simulink model "fullSystemModel"  (R2018a)
settings: Solver=ode3  StartTime=0.0  StopTime=1000  FixedStep=1  MinStep=1e-8  RelTol=1e-8
undefined symbols (not defined in the file or in its folder): DiscIntNeverNeededParam
libraries: BupSimulinkLibraries x32, simulink_extras x22, simulink x2, SignalEditorBlockLib x2
(part 1 of 3)
settings Model: PauseTimes=500  PacingRate=5  Creator=Юзер33  LastModifiedBy=User33
settings DataIOCC: SaveFormat=Array  OutputSaveName=P_lon
settings OptimizationCC: DefaultParameterBehavior=Inlined  UseDivisionForNetSlopeComputation=on  UseFloatMulNetSlope=on  InlineInvariantSignals=on  PassReuseOutputArgsAs=Individual arguments  ZeroExternalMemoryAtStartup=off  ZeroInternalMemoryAtStartup=off  NoFixptDivByZeroProtection=on  EfficientFloat2IntCast=on  LifeSpan=1  OptimizationLevel=level1  OptimizationCustomize=off
settings DebuggingCC: ParameterTunabilityLossMsg=error
settings HardwareCC: ProdBitPerPointer=32  ProdBitPerSizeT=32  ProdBitPerPtrDiffT=32  ProdLargestAtomicInteger=Long  ProdLargestAtomicFloat=Double  ProdWordSize=32  ProdHWDeviceType=ARM Compatible->ARM Cortex
settings SFSimCC: MATLABDynamicMemAlloc=off
settings RTWCC: SystemTargetFile=ert.tlc  GenCodeOnly=on  PackageGeneratedCodeAndArtifacts=on  PackageName=BupModel  TemplateMakefile=ert_default_tmf  GenerateReport=on  RTWVerbose=off  RTWUseSimCustomCode=on  BuildConfiguration=Faster Runs  IncludeHyperlinkInReport=on  LaunchReport=on  GenerateTraceInfo=on  GenerateTraceReport=on  GenerateTraceReportSl=on  GenerateTraceReportSf=on  GenerateTraceReportEml=on  GenerateWebview=on  GenerateCodeMetricsReport=on  GenerateCodeReplacementReport=on
settings CodeAppCC: ForceParamTrailComments=on  IgnoreCustomStorageClasses=off  OperatorAnnotations=on  SimulinkDataObjDesc=on  SFDataObjDesc=on  MATLABFcnDesc=on  CustomSymbolStrGlobalVar=rt$N$M  CustomSymbolStrType=$N$M  CustomSymbolStrFcn=$N$M$F  CustomSymbolStrMacro=$N$M  InsertBlockDesc=on  StateflowObjectComments=on  MATLABSourceComments=on  ReqsInCode=on  UseSimReservedNames=on
settings ERTTargetCC: TargetLangStandard=C99 (ISO)  GenerateSampleERTMain=on  IncludeMdlTerminateFcn=off  CombineSignalStateStructs=on  SupportComplex=off  SupportNonInlinedSFcns=on  RemoveResetFunc=off  InlinedParameterPlacement=NonHierarchical  RootIOFormat=Structure reference  ERTCustomFileTemplate=example_file_process.tlc  ERTFilePackagingFormat=CompactWithDataFile  IndentStyle=Allman

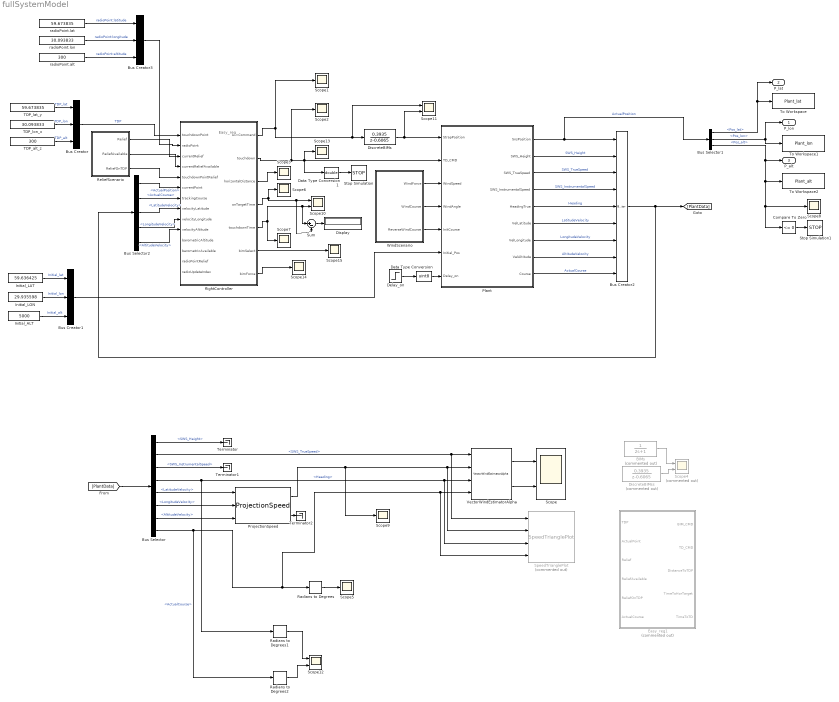
== system fullSystemModel ==
  note: Easy_reg_
  BIMs : TransferFcn  Commented=on  Denominator=[2 1]
  Bus Creator : BusCreator  Inputs=3
  Bus Creator1 : BusCreator  Inputs=3
  Bus Creator2 : BusCreator  Inputs=9
  Bus Creator3 : BusCreator  Inputs=3
  Bus Selector : BusSelector  OutputSignals=SWS_Height,SWS_TrueSpeed,SWS_InstrumentalSpeed,Heading,LatitudeVelocity,LongitudeVelocity,AltitudeVelocity,ActualCourse
  Bus Selector1 : BusSelector  OutputSignals=Pos_lat,Pos_lon,Pos_alt
  Bus Selector2 : BusSelector  OutputSignals=ActualPosition,ActualCourse,LatitudeVelocity,LongitudeVelocity,AltitudeVelocity
  Compare To Zero : simulink/Logic and Bit Operations/Compare To Zero  relop=<=  OutDataTypeStr=boolean
  Data Type Conversion : DataTypeConversion  OutDataTypeStr=uint8
  Data Type Conversion1 : DataTypeConversion  OutDataTypeStr=double
  Delay_on : Step  Time=20  Before=1  SampleTime=0
  DiscreteBIMs : DiscreteTransferFcn  Numerator=[0.3935]  Denominator=[1 -0.6065]
  DiscreteBIMss : DiscreteTransferFcn  Commented=on  Numerator=[0.3935]  Denominator=[1 -0.6065]
  Display : Display
  Easy_reg1 : Subsystem  Commented=on  TreatAsAtomicUnit=on  SystemSampleTime=1
  Initial_ALT : Constant  Value=5000
  Initial_LAT : Constant  Value=59.636425
  Initial_LON : Constant  Value=29.935598
  Plant : Subsystem  TreatAsAtomicUnit=on
  ProjectionSpeed : BupSimulinkLibraries/ProjectionSpeed
  Radians to Degrees : simulink_extras/Transformations/Radians to Degrees
  Radians to Degrees1 : simulink_extras/Transformations/Radians to Degrees
  Radians to Degrees2 : simulink_extras/Transformations/Radians to Degrees
  ReliefScenario : Subsystem  SystemSampleTime=1
  Scope{,10..12} (4 alike) : Scope  NumInputPorts=2
  Scope{1..3,5..9,13..15} (11 alike) : Scope
  Scope4 : Scope  Commented=on  NumInputPorts=2
  SpeedTrianglePlot : BupSimulinkLibraries/SpeedTrianglePlot  Commented=on
  Stop Simulation : Stop
  Stop Simulation1 : Stop
  Sum : Sum  Inputs=|+-
  TDP_alt_z : Constant  Value=300
  TDP_lat_y : Constant  Value=59.673835
  TDP_lon_x : Constant  Value=30.093833
  Terminator : Terminator
  Terminator1 : Terminator
  Terminator2 : Terminator
  To Workspace : ToWorkspace  VariableName=Plant_lat  SaveFormat=Timeseries  SampleTime=-1
  To Workspace1 : ToWorkspace  VariableName=Plant_lon  SaveFormat=Timeseries  SampleTime=-1
  To Workspace2 : ToWorkspace  VariableName=Plant_alt  SaveFormat=Timeseries  SampleTime=-1
  VectorWindEstimatorAlpha : BupSimulinkLibraries/VectorWindEstimatorAlpha  SystemSampleTime=-1
  WindScenario : Subsystem  SystemSampleTime=1
  flightController : Subsystem  TreatAsAtomicUnit=on  SystemSampleTime=1
  radioPoint.alt : Constant  Value=300
  radioPoint.lat : Constant  Value=59.673835
  radioPoint.lon : Constant  Value=30.093833
  P_lon : Outport
  P_lat : Outport  Port=2
  P_alt : Outport  Port=3
  wires:
  TDP_alt_z/1 -> Bus Creator/3  "TDP_alt"
  TDP_lon_x/1 -> Bus Creator/2  "TDP_lon"
  TDP_lat_y/1 -> Bus Creator/1  "TDP_lat"
  Bus Creator/1 -> flightController/1(touchdownPoint)  "TDP"
  Plant/1(SnsPosition) -> Bus Creator2/1, Bus Selector1/1  "ActualPosition"
  Initial_LAT/1 -> Bus Creator1/1  "Initial_lat"
  Initial_LON/1 -> Bus Creator1/2  "Initial_lon"
  Initial_ALT/1 -> Bus Creator1/3  "Initial_alt"
  BIMs/1 -> Scope4/1
  DiscreteBIMss/1 -> Scope4/2
  Bus Selector1/1 -> To Workspace/1, P_lat/1  "<Pos_lat>"
  Delay_on/1 -> Data Type Conversion/1
  DiscreteBIMs/1 -> Plant/1(StrapPosition), Scope11/2
  flightController/1(bimCommand) -> Scope1/1, Scope11/1, DiscreteBIMs/1
  flightController/2(touchdown) -> Scope2/1, Scope13/1, Data Type Conversion1/1, Plant/2(TD_CMD)
  Data Type Conversion/1 -> Plant/7(Delay_on)
  Bus Selector1/2 -> P_lon/1, To Workspace1/1  "<Pos_lon>"
  Bus Selector1/3 -> Scope8/1, Compare To Zero/1, To Workspace2/1, P_alt/1  "<Pos_alt>"
  Plant/7(VelLongitude) -> Bus Creator2/7  "LongitudeVelocity"
  Plant/8(VelAltitude) -> Bus Creator2/8  "AltitudeVelocity"
  Plant/6(VelLatitude) -> Bus Creator2/6  "LatitudeVelocity"
  Plant/2(SWS_Height) -> Bus Creator2/2  "SWS_Height"
  Plant/5(HeadingTrue) -> Bus Creator2/5  "Heading"
  Plant/4(SWS_InstrumentalSpeed) -> Bus Creator2/4  "SWS_InstrumentalSpeed"
  Plant/9(Course) -> Bus Creator2/9  "ActualCourse"
  Plant/3(SWS_TrueSpeed) -> Bus Creator2/3  "SWS_TrueSpeed"
  WindScenario/2(WindCourse) -> Plant/4(WindAngle)
  WindScenario/1(WindForce) -> Plant/3(WindSpeed)
  WindScenario/3(ReverseWindCourse) -> Plant/5(InitCourse)
  [PlantData] -> Bus Selector/1
  Bus Selector/6 -> ProjectionSpeed/2  "<LongitudeVelocity>"
  Bus Selector/2 -> SpeedTrianglePlot/1, VectorWindEstimatorAlpha/1  "<SWS_TrueSpeed>"
  Radians to Degrees/1 -> Scope5/1
  Bus Selector/8 -> Radians to Degrees2/1, SpeedTrianglePlot/4, VectorWindEstimatorAlpha/4, Radians to Degrees/1  "<ActualCourse>"
  Bus Selector/4 -> Radians to Degrees1/1, SpeedTrianglePlot/3, VectorWindEstimatorAlpha/3  "<Heading>"
  VectorWindEstimatorAlpha/1 -> Scope/1
  VectorWindEstimatorAlpha/2 -> Scope/2
  ProjectionSpeed/1 -> Scope9/1, SpeedTrianglePlot/2, VectorWindEstimatorAlpha/2
  Bus Selector/5 -> ProjectionSpeed/1  "<LatitudeVelocity>"
  Bus Selector/7 -> ProjectionSpeed/3  "<AltitudeVelocity>"
  Data Type Conversion1/1 -> Stop Simulation/1
  flightController/3(horizontalDistance) -> Scope3/1
  Compare To Zero/1 -> Stop Simulation1/1
  ReliefScenario/1(Relief) -> flightController/3(currentRelief)
  ReliefScenario/2(ReliefAvailable) -> flightController/4(currentReliefAvailable)
  ReliefScenario/3(ReliefOnTDP) -> flightController/5(touchdownPointRelief)
  Bus Creator2/1 -> Bus Selector2/1, [PlantData]
  Bus Selector2/1 -> flightController/6(currentPoint)  "<ActualPosition>"
  Bus Selector2/2 -> flightController/7(trackingCourse)  "<ActualCourse>"
  Bus Selector2/3 -> flightController/8(velocityLatitude)  "<LatitudeVelocity>"
  Bus Selector2/4 -> flightController/9(velocityLongitude)  "<LongitudeVelocity>"
  Bus Selector2/5 -> flightController/10(velocityAltitude)  "<AltitudeVelocity>"
  Bus Creator1/1 -> Plant/6(Initial_Pos)
  flightController/5(touchdownTime) -> Sum/1, Scope10/2, Scope7/1
  flightController/4(onTargetTime) -> Scope6/1, Sum/2, Scope10/1
  Bus Selector/1 -> Terminator/1  "<SWS_Height>"
  Bus Selector/3 -> Terminator1/1  "<SWS_InstrumentalSpeed>"
  ProjectionSpeed/2 -> Terminator2/1
  Sum/1 -> Display/1
  Radians to Degrees1/1 -> Scope12/1
  Radians to Degrees2/1 -> Scope12/2
  flightController/7(bimForce) -> Scope14/1
  flightController/6(bimSelect) -> Scope15/1
  radioPoint.lon/1 -> Bus Creator3/2  "radioPoint:longitude"
  radioPoint.alt/1 -> Bus Creator3/3  "radioPoint:altitude"
  radioPoint.lat/1 -> Bus Creator3/1  "radioPoint:latitude"
  Bus Creator3/1 -> flightController/2(radioPoint)

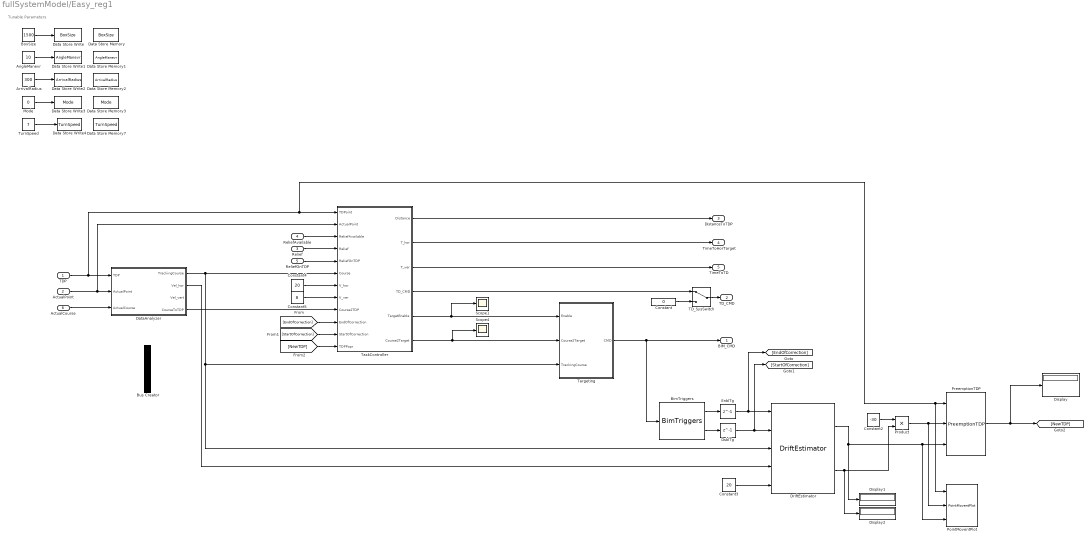
== system fullSystemModel/Easy_reg1 ==
  note: Tunable Parameters
  TDP : Inport
  ActualPoint : Inport  Port=2
  Relief : Inport  Port=3
  ReliefAvailable : Inport  Port=4
  ReliefOnTDP : Inport  Port=5
  ActualCourse : Inport  Port=6
  AngleManevr : Constant  Value=10
  ArrivalRadius : Constant  Value=300
  BimTriggers : BupSimulinkLibraries/BimTriggers
  BoxSize : Constant  Value=1500
  Bus Creator : BusCreator  Inputs=6
  Constant : Constant  Value=0
  Constant2 : Constant  Value=-30
  Constant3 : Constant  Value=20
  Constant4 : Constant  Value=20
  Constant5 : Constant  Value=8
  Data Store Memory : DataStoreMemory  DataStoreName=BoxSize  ReadBeforeWriteMsg=warning  WriteAfterWriteMsg=warning  WriteAfterReadMsg=warning  ShowAdditionalParam=off  OutDataTypeStr=double  Dimensions=1
  Data Store Memory1 : DataStoreMemory  DataStoreName=AngleManevr  ReadBeforeWriteMsg=warning  WriteAfterWriteMsg=warning  WriteAfterReadMsg=warning  ShowAdditionalParam=off  OutDataTypeStr=double  Dimensions=1
  Data Store Memory2 : DataStoreMemory  DataStoreName=ArrivalRadius  ReadBeforeWriteMsg=warning  WriteAfterWriteMsg=warning  WriteAfterReadMsg=warning  ShowAdditionalParam=off  OutDataTypeStr=double  Dimensions=1
  Data Store Memory3 : DataStoreMemory  DataStoreName=Mode  ReadBeforeWriteMsg=warning  WriteAfterWriteMsg=warning  WriteAfterReadMsg=warning  ShowAdditionalParam=off  OutDataTypeStr=uint8  Dimensions=1
  Data Store Memory7 : DataStoreMemory  DataStoreName=TurnSpeed  ReadBeforeWriteMsg=warning  WriteAfterWriteMsg=warning  WriteAfterReadMsg=warning  ShowAdditionalParam=off  OutDataTypeStr=double  Dimensions=1
  Data Store Write : DataStoreWrite  DataStoreName=BoxSize
  Data Store Write1 : DataStoreWrite  DataStoreName=AngleManevr
  Data Store Write2 : DataStoreWrite  DataStoreName=ArrivalRadius
  Data Store Write3 : DataStoreWrite  DataStoreName=Mode
  Data Store Write4 : DataStoreWrite  DataStoreName=TurnSpeed
  DataAnalyzer : Subsystem
  Display : Display
  Display1 : Display
  Display2 : Display
  DriftEstimator : BupSimulinkLibraries/DriftEstimator
  DsblTg : Delay  DelayLength=1  InitialCondition=0
  EnblTg : Delay  DelayLength=1  InitialCondition=0
  Mode : Constant  Value=0  OutDataTypeStr=uint8
  PointMoventPlot : BupSimulinkLibraries/PointMoventPlot
  PreemptionTDP : BupSimulinkLibraries/PreemptionTDP
  Product : Product
  Scope1 : Scope
  Scope4 : Scope
  TD_SysSwitch : ManualSwitch
  Targeting : Subsystem
  TaskController : Stateflow chart  TreatAsAtomicUnit=on  SystemSampleTime=1
  TurnSpeed : Constant  Value=7  OutDataTypeStr=double
  BIM_CMD : Outport
  TD_CMD : Outport  Port=2  OutDataTypeStr=uint8
  DistanceToTDP : Outport  Port=3
  TimeToHorTarget : Outport  Port=4
  TimeToTD : Outport  Port=5
  wires:
  TaskController/4(TD_CMD) -> TD_SysSwitch/1
  BoxSize/1 -> Data Store Write/1
  AngleManevr/1 -> Data Store Write1/1
  ArrivalRadius/1 -> Data Store Write2/1
  TD_SysSwitch/1 -> TD_CMD/1
  Constant/1 -> TD_SysSwitch/2
  Mode/1 -> Data Store Write3/1
  TurnSpeed/1 -> Data Store Write4/1
  TaskController/5(TargetEnable) -> Scope1/1, Targeting/1(Enable)
  DataAnalyzer/2(Vel_hor) -> DriftEstimator/4
  ActualCourse/1 -> DataAnalyzer/3(ActualCourse)
  ReliefAvailable/1 -> TaskController/3(ReliefAvailable)
  Relief/1 -> TaskController/4(Relief)
  ReliefOnTDP/1 -> TaskController/5(ReliefOnTDP)
  TaskController/1(Distance) -> DistanceToTDP/1
  TaskController/2(T_hor) -> TimeToHorTarget/1
  TaskController/3(T_ver) -> TimeToTD/1
  ActualPoint/1 -> DataAnalyzer/2(ActualPoint), TaskController/2(ActualPoint)
  TaskController/6(Course2Target) -> Targeting/2(Course2Target), Scope4/1
  Targeting/1(CMD) -> BimTriggers/1, BIM_CMD/1
  BimTriggers/2 -> DsblTg/1
  DataAnalyzer/1(TrackingCourse) -> DriftEstimator/3, Targeting/3(TrackingCourse), TaskController/6(Course)
  DataAnalyzer/4(CourseToTDP) -> TaskController/9(Course2TDP)
  BimTriggers/1 -> EnblTg/1
  Constant2/1 -> Product/1
  TDP/1 -> PointMoventPlot/1, PreemptionTDP/1, TaskController/1(TDPoint), DataAnalyzer/1(TDP)
  Product/1 -> PointMoventPlot/2, PreemptionTDP/2
  DriftEstimator/2 -> Display2/1, Product/2
  DriftEstimator/1 -> Display1/1, PointMoventPlot/3, PreemptionTDP/3
  EnblTg/1 -> [EndOfCorrection], DriftEstimator/1
  DsblTg/1 -> [StartOfCorrection], DriftEstimator/2
  Constant3/1 -> DriftEstimator/5
  Constant5/1 -> TaskController/8(V_ver)
  Constant4/1 -> TaskController/7(V_hor)
  PreemptionTDP/1 -> [NewTDP], Display/1
  [EndOfCorrection] -> TaskController/10(EndOfCorrection)
  [NewTDP] -> TaskController/12(TDPPopr)
  [StartOfCorrection] -> TaskController/11(StartOfCorrection)

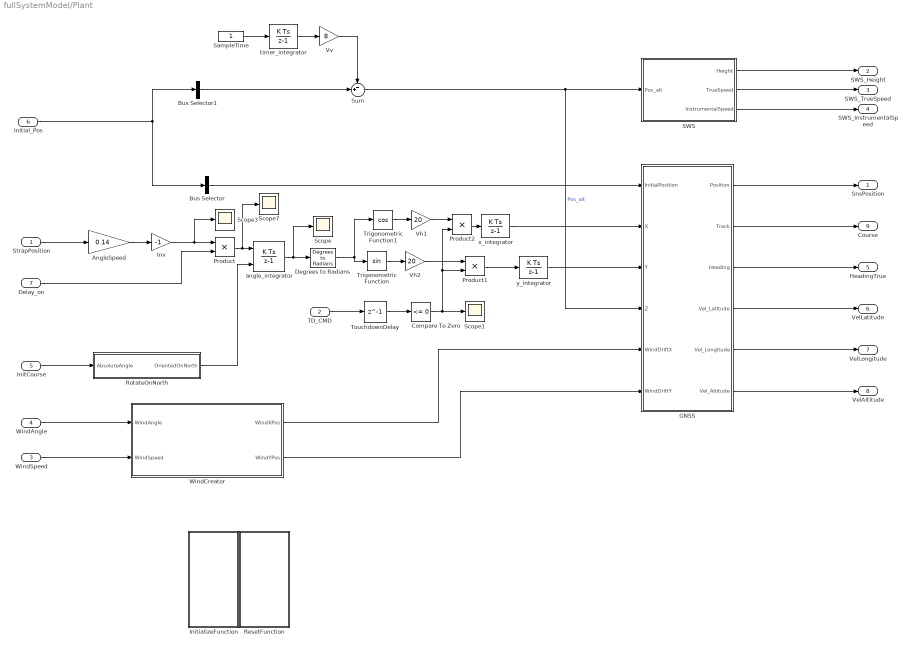
== system fullSystemModel/Plant ==
  StrapPosition : Inport  OutDataTypeStr=double  PortDimensions=1
  TD_CMD : Inport  Port=2  OutDataTypeStr=uint8  PortDimensions=1
  WindSpeed : Inport  Port=3
  WindAngle : Inport  Port=4
  InitCourse : Inport  Port=5
  Initial_Pos : Inport  Port=6
  Delay_on : Inport  Port=7
  AngleSpeed : Gain  Gain=0.14
  Bus Selector : BusSelector  OutputSignals=Initial_lat,Initial_lon  OutputAsBus=on
  Bus Selector1 : BusSelector  OutputSignals=Initial_alt  OutputAsBus=on
  Compare To Zero : simulink/Logic and Bit Operations/Compare To Zero  relop=<=  OutDataTypeStr=boolean
  Degrees to Radians : simulink_extras/Transformations/Degrees to Radians
  GNSS : Subsystem
  InitializeFunction : Subsystem  TreatAsAtomicUnit=on
  Inv : Gain  Gain=-1
  Product : Product
  Product1 : Product
  Product2 : Product
  ResetFunction : Subsystem  TreatAsAtomicUnit=on
  RotateOnNorth : Subsystem
  SWS : Subsystem
  SampleTime : Constant
  Scope{,1,3,7} (4 alike) : Scope
  Sum : Sum  Inputs=-+|
  TouchdownDelay : Delay  DelayLength=1  InitialCondition=0
  Trigonometric Function : Trigonometry
  Trigonometric Function1 : Trigonometry  Operator=cos
  Vh1 : Gain  Gain=20
  Vh2 : Gain  Gain=20
  Vv : Gain  Gain=8
  WindCreator : Subsystem
  angle_integrator : DiscreteIntegrator  InitialConditionSource=external  InitialCondition=90  SampleTime=-1  ICPrevOutput=DiscIntNeverNeededParam  ICPrevScaledInput=DiscIntNeverNeededParam
  timer_integrator : DiscreteIntegrator  SampleTime=-1  ICPrevOutput=DiscIntNeverNeededParam  ICPrevScaledInput=DiscIntNeverNeededParam
  x_integrator : DiscreteIntegrator  SampleTime=-1  ICPrevOutput=DiscIntNeverNeededParam  ICPrevScaledInput=DiscIntNeverNeededParam
  y_integrator : DiscreteIntegrator  SampleTime=-1  ICPrevOutput=DiscIntNeverNeededParam  ICPrevScaledInput=DiscIntNeverNeededParam
  SnsPosition : Outport
  SWS_Height : Outport  Port=2
  SWS_TrueSpeed : Outport  Port=3
  SWS_InstrumentalSpeed : Outport  Port=4
  HeadingTrue : Outport  Port=5
  VelLatitude : Outport  Port=6
  VelLongitude : Outport  Port=7
  VelAltitude : Outport  Port=8
  Course : Outport  Port=9
  wires:
  Degrees to Radians/1 -> Trigonometric Function1/1, Trigonometric Function/1
  angle_integrator/1 -> Scope/1, Degrees to Radians/1
  Trigonometric Function1/1 -> Vh1/1
  Trigonometric Function/1 -> Vh2/1
  Inv/1 -> Product/1, Scope3/1
  Delay_on/1 -> Product/2
  timer_integrator/1 -> Vv/1
  Vv/1 -> Sum/1
  Sum/1 -> GNSS/4(Z), SWS/1(Pos_alt)  "Pos_alt"
  Initial_Pos/1 -> Bus Selector1/1, Bus Selector/1
  Bus Selector/1 -> GNSS/1(InitialPosition)
  Bus Selector1/1 -> Sum/2
  StrapPosition/1 -> AngleSpeed/1
  Product/1 -> Scope7/1, angle_integrator/1
  AngleSpeed/1 -> Inv/1
  SWS/1(Height) -> SWS_Height/1
  SWS/2(TrueSpeed) -> SWS_TrueSpeed/1
  SWS/3(InstrumentalSpeed) -> SWS_InstrumentalSpeed/1
  SampleTime/1 -> timer_integrator/1
  InitCourse/1 -> RotateOnNorth/1(AbsoluteAngle)
  TD_CMD/1 -> TouchdownDelay/1
  WindAngle/1 -> WindCreator/1(WindAngle)
  WindSpeed/1 -> WindCreator/2(WindSpeed)
  RotateOnNorth/1(OrientedOnNorth) -> angle_integrator/2
  x_integrator/1 -> GNSS/2(X)
  y_integrator/1 -> GNSS/3(Y)
  WindCreator/1(WindXPos) -> GNSS/5(WindDriftX)
  WindCreator/2(WindYPos) -> GNSS/6(WindDriftY)
  GNSS/1(Position) -> SnsPosition/1
  GNSS/3(Heading) -> HeadingTrue/1
  GNSS/2(Track) -> Course/1
  GNSS/4(Vel_Latitude) -> VelLatitude/1
  GNSS/5(Vel_Longitude) -> VelLongitude/1
  GNSS/6(Vel_Altitude) -> VelAltitude/1
  Vh1/1 -> Product2/1
  Vh2/1 -> Product1/1
  TouchdownDelay/1 -> Compare To Zero/1
  Compare To Zero/1 -> Product2/2, Product1/2, Scope1/1
  Product1/1 -> y_integrator/1
  Product2/1 -> x_integrator/1

== system fullSystemModel/ReliefScenario ==
  AutoModeA : ManualSwitch  CurrentSetting=0
  AutoModeR : ManualSwitch  CurrentSetting=0
  ReliefAvailableValue : Constant  OutDataTypeStr=uint8
  ReliefOnTDPValue : Constant  Value=100  OutDataTypeStr=int16
  ReliefValue : Constant  Value=100  OutDataTypeStr=int16
  Scope{,1..3} (4 alike) : Scope
  SignalEditor : SignalEditorBlockLib/Signal Editor  FileName=ReliefScenario.mat  ActiveScenario=Scenario  ActiveSignal=ReliefAvailable  IsBus=off  OutputBusObjectStr=Bus: BusObject  SampleTime=1  Interpolate=off  ZeroCross=off  OutputAfterFinalValue=Setting to zero  Unit=inherit
  Relief : Outport
  ReliefAvailable : Outport  Port=2
  ReliefOnTDP : Outport  Port=3
  wires:
  SignalEditor/2 -> Scope1/1, AutoModeA/1
  SignalEditor/1 -> Scope/1, AutoModeR/1
  ReliefAvailableValue/1 -> AutoModeA/2
  ReliefValue/1 -> AutoModeR/2
  AutoModeR/1 -> Scope2/1, Relief/1
  AutoModeA/1 -> Scope3/1, ReliefAvailable/1
  ReliefOnTDPValue/1 -> ReliefOnTDP/1

== system fullSystemModel/WindScenario ==
  AutoModeA : ManualSwitch
  AutoModeS : ManualSwitch
  Constant : Constant  Value=180
  Constant1 : Constant  Value=0
  Degrees to Radians : simulink_extras/Transformations/Degrees to Radians
  Manual Switch : ManualSwitch  CurrentSetting=0
  Scope1 : Scope
  Scope2 : Scope
  Scope3 : Scope
  SignalEditor : SignalEditorBlockLib/Signal Editor  FileName=WindScenario.mat  ActiveScenario=Scenario  ActiveSignal=WindHeading  IsBus=off  OutputBusObjectStr=Bus: BusObject  SampleTime=1  ZeroCross=off  OutputAfterFinalValue=Setting to zero  Unit=inherit
  Sum : Sum  Inputs=++|
  WindAngle : Constant  Value=0
  WindSpeed : Constant  Value=0
  WindForce : Outport
  WindCourse : Outport  Port=2
  ReverseWindCourse : Outport  Port=3
  wires:
  SignalEditor/1 -> AutoModeS/1, Scope2/1
  WindAngle/1 -> AutoModeA/2
  WindSpeed/1 -> AutoModeS/2
  AutoModeS/1 -> WindForce/1
  AutoModeA/1 -> WindCourse/1, Sum/2
  Sum/1 -> Manual Switch/1
  Constant/1 -> Sum/1
  Manual Switch/1 -> ReverseWindCourse/1
  Constant1/1 -> Manual Switch/2
  SignalEditor/2 -> AutoModeA/1, Scope3/1, Degrees to Radians/1
  Degrees to Radians/1 -> Scope1/1

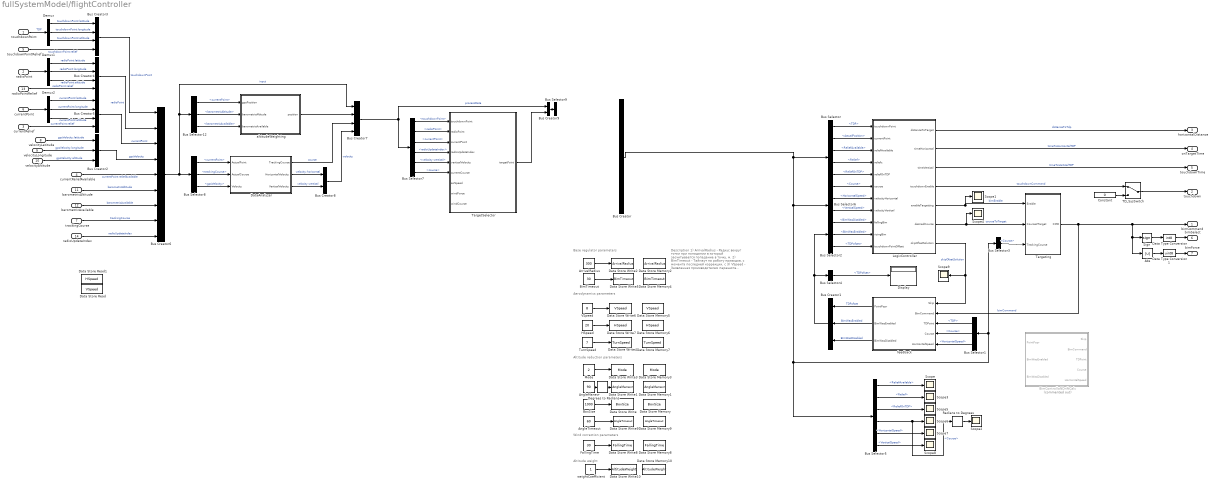
== system fullSystemModel/flightController ==
  note: Altitude weight
  note: Description
      | 1) ArrivalRadius - Радиус вокруг
      | точки при попадании в который
      | засчитывается попадание в
      | точку, м.
      | 2) BimTimeout - Таймаут на работу
      | приводов, с момента последней
      | коррекции, с
      |
      |
      | 3) VSpeed - Заявленная
      | производителем парашюта
      | вертикальная скорость снижения
      | парашюта, м/с.
      | 4) HSpeed - Заявленная
      | производителем парашюта
      | горизонтальная скорость движения
      | парашюта, м/с.
      | 5) TurnSpeed - Заявленная
      | производителем парашюта
      | скорость разворота при 50%
      | затяжке стропы, град/с.
      |
      |
      | 6) Mode - Режим работы
      | регулятора.
      |
      | 7) AngleManevr - Угол отклонения
      | от заданного курса при работе
      | регулятора в
      | режиме углового манёвра, град.
      |
      | 8) BoxSize - Размер коробки в
      | режиме работы 1-Box, м.
      |
      | 9) AngleTimeout - Таймаут между
      | шагами алгоритма потери высоты
      | в режиме работы 3-Angle, сек.
      |
      | 10) FallingTime - Расчетное время
      | между введением посадочной
      | системы в действие и посадкой,
      | сек.
      |
      | 11) Весовой коэффициент
      | для определения высоты (0...1):
      | = 1 Если доверяем только высоте
      | со спутника;
      | = 0 Если доверяем только
      | барометрической высоте;
  note: Altitude reduction parameters
  note: Aerodynamics parameters
  note: Base regulator parameters
  note: Wind correction parameters
  touchdownPoint : Inport
  radioPoint : Inport  Port=2  PortDimensions=3
  currentRelief : Inport  Port=3
  currentReliefAvailable : Inport  Port=4
  touchdownPointRelief : Inport  Port=5
  currentPoint : Inport  Port=6
  trackingCourse : Inport  Port=7
  velocityLatitude : Inport  Port=8
  velocityLongitude : Inport  Port=9
  velocityAltitude : Inport  Port=10
  barometricAltitude : Inport  Port=11
  barometricAvailable : Inport  Port=12
  radioPointRelief : Inport  Port=13
  radioUpdateIndex : Inport  Port=14
  Abs : Abs
  AngleManevr : Constant  Value=90
  AngleTimeout : Constant  Value=60  OutDataTypeStr=uint32
  ArrivalRadius : Constant  Value=300
  BimControllaNDriftCalc : Subsystem  Commented=on
  BimTimeout : Constant  Value=30  OutDataTypeStr=uint32
  BoxSize : Constant  Value=1000
  Bus Creator : BusCreator  Inputs=10
  Bus Creator1 : BusCreator  Inputs=3
  Bus Creator2 : BusCreator  Inputs=3
  Bus Creator{3..5,7} (4 alike) : BusCreator  Inputs=4
  Bus Creator6 : BusCreator  Inputs=9
  Bus Creator8 : BusCreator  Inputs=2
  Bus Creator9 : BusCreator  Inputs=2
  Bus Selector : BusSelector  OutputSignals=TDP,ActualPosition,ReliefAvailable,Relief,ReliefOnTDP,Course
  Bus Selector1 : BusSelector  OutputSignals=TDP,Course,HorizontalSpeed
  Bus Selector12 : BusSelector  OutputSignals=currentPoint,barometricAltitude,barometricAvailable
  Bus Selector2 : BusSelector  OutputSignals=BimWasDisabled,BimWasEnabled,TDPofset
  Bus Selector3 : BusSelector  OutputSignals=Course
  Bus Selector4 : BusSelector  OutputSignals=TDPofset
  Bus Selector5 : BusSelector  OutputSignals=ReliefAvailable,Relief,ReliefOnTDP,Course,HorizontalSpeed,VerticalSpeed
  Bus Selector6 : BusSelector  OutputSignals=HorizontalSpeed,VerticalSpeed
  Bus Selector7 : BusSelector  OutputSignals=input.touchdownPoint,input.radioPoint,currentPoint,input.radioUpdateIndex,velocity.velocity:vertical,course
  Bus Selector8 : BusSelector  OutputSignals=currentPoint,trackingCourse,gpsVelocity
  Bus Selector9 : BusSelector  OutputSignals=processData.currentPoint,targetPoint,processData.course,processData.velocity,processData.input.currentPoint:reliefAvailable  OutputAsBus=on
  Constant : Constant  Value=0
  Data Store Memory : DataStoreMemory  DataStoreName=BoxSize  ReadBeforeWriteMsg=warning  WriteAfterWriteMsg=warning  WriteAfterReadMsg=warning  ShowAdditionalParam=off  OutDataTypeStr=double  Dimensions=1
  Data Store Memory1 : DataStoreMemory  DataStoreName=AngleManevr  ReadBeforeWriteMsg=warning  WriteAfterWriteMsg=warning  WriteAfterReadMsg=warning  ShowAdditionalParam=off  OutDataTypeStr=double  Dimensions=1
  Data Store Memory10 : DataStoreMemory  DataStoreName=AltitudeWeight  ReadBeforeWriteMsg=warning  WriteAfterWriteMsg=warning  WriteAfterReadMsg=warning  ShowAdditionalParam=off  OutDataTypeStr=double  Dimensions=1
  Data Store Memory2 : DataStoreMemory  DataStoreName=ArrivalRadius  ReadBeforeWriteMsg=warning  WriteAfterWriteMsg=warning  WriteAfterReadMsg=warning  ShowAdditionalParam=off  OutDataTypeStr=double  Dimensions=1
  Data Store Memory3 : DataStoreMemory  DataStoreName=Mode  ReadBeforeWriteMsg=warning  WriteAfterWriteMsg=warning  WriteAfterReadMsg=warning  ShowAdditionalParam=off  OutDataTypeStr=uint8  Dimensions=1
  Data Store Memory4 : DataStoreMemory  DataStoreName=BimTimeout  ReadBeforeWriteMsg=warning  WriteAfterWriteMsg=warning  WriteAfterReadMsg=warning  ShowAdditionalParam=off  OutDataTypeStr=uint32  Dimensions=1
  Data Store Memory5 : DataStoreMemory  DataStoreName=VSpeed  ReadBeforeWriteMsg=warning  WriteAfterWriteMsg=warning  WriteAfterReadMsg=warning  ShowAdditionalParam=off  OutDataTypeStr=double  Dimensions=1
  Data Store Memory6 : DataStoreMemory  DataStoreName=HSpeed  ReadBeforeWriteMsg=warning  WriteAfterWriteMsg=warning  WriteAfterReadMsg=warning  ShowAdditionalParam=off  OutDataTypeStr=double  Dimensions=1
  Data Store Memory7 : DataStoreMemory  DataStoreName=TurnSpeed  ReadBeforeWriteMsg=warning  WriteAfterWriteMsg=warning  WriteAfterReadMsg=warning  ShowAdditionalParam=off  OutDataTypeStr=double  Dimensions=1
  Data Store Memory8 : DataStoreMemory  DataStoreName=FallingTime  ReadBeforeWriteMsg=warning  WriteAfterWriteMsg=warning  WriteAfterReadMsg=warning  ShowAdditionalParam=off  OutDataTypeStr=double  Dimensions=1
  Data Store Memory9 : DataStoreMemory  DataStoreName=AngleTimeout  ReadBeforeWriteMsg=warning  WriteAfterWriteMsg=warning  WriteAfterReadMsg=warning  ShowAdditionalParam=off  OutDataTypeStr=uint32  Dimensions=1
  Data Store Read : DataStoreRead  DataStoreName=VSpeed
  Data Store Read1 : DataStoreRead  DataStoreName=HSpeed
  Data Store Write : DataStoreWrite  DataStoreName=BoxSize
  Data Store Write1 : DataStoreWrite  DataStoreName=AngleManevr
  Data Store Write10 : DataStoreWrite  DataStoreName=AltitudeWeight
  Data Store Write2 : DataStoreWrite  DataStoreName=ArrivalRadius
  Data Store Write3 : DataStoreWrite  DataStoreName=Mode
  Data Store Write4 : DataStoreWrite  DataStoreName=TurnSpeed
  Data Store Write5 : DataStoreWrite  DataStoreName=BimTimeout
  Data Store Write6 : DataStoreWrite  DataStoreName=VSpeed
  Data Store Write7 : DataStoreWrite  DataStoreName=HSpeed
  Data Store Write8 : DataStoreWrite  DataStoreName=FallingTime
  Data Store Write9 : DataStoreWrite  DataStoreName=AngleTimeout
  Data Type Conversion : DataTypeConversion  OutDataTypeStr=int8
  Data Type Conversion1 : DataTypeConversion  OutDataTypeStr=uint8
  DataAnalyzer : Subsystem
  Degrees to Radians : simulink_extras/Transformations/Degrees to Radians
  Demux : Demux  Outputs=3
  Demux1 : Demux  Outputs=3
  Demux2 : Demux  Outputs=3
  Display : Display
  FallingTime : Constant  Value=30
  HSpeed : Constant  Value=20
  LogicController : Stateflow chart  TreatAsAtomicUnit=on  SystemSampleTime=1
  Mode : Constant  Value=2  OutDataTypeStr=uint8
  Radians to Degrees : simulink_extras/Transformations/Radians to Degrees
  Scope{,1..9} (10 alike) : Scope
  Sign : Signum
  TD_SysSwitch : ManualSwitch
  TargetSelector : Stateflow chart  TreatAsAtomicUnit=on
  Targeting : Subsystem
  TurnSpeed : Constant  Value=7  OutDataTypeStr=double
  VSpeed : Constant  Value=8
  altitudeWeighting : Subsystem
  feedback : Subsystem
  weightCoefficient : Constant  OutMin=[0]  OutMax=[1]  OutDataTypeStr=double
  bimCommand : Outport
  touchdown : Outport  Port=2  OutDataTypeStr=uint8
  horizontalDistance : Outport  Port=3
  onTargetTime : Outport  Port=4
  touchdownTime : Outport  Port=5
  bimSelect : Outport  Port=6  OutDataTypeStr=int8
  bimForce : Outport  Port=7  OutDataTypeStr=uint8
  wires:
  LogicController/4(touchdownEnable) -> TD_SysSwitch/1  "touchdownCommand"
  BoxSize/1 -> Data Store Write/1
  AngleManevr/1 -> Degrees to Radians/1
  ArrivalRadius/1 -> Data Store Write2/1
  TD_SysSwitch/1 -> touchdown/1
  Constant/1 -> TD_SysSwitch/2
  Mode/1 -> Data Store Write3/1
  TurnSpeed/1 -> Data Store Write4/1
  LogicController/5(enableTargetting) -> Scope1/1, Targeting/1(Enable)  "bimEnable"
  LogicController/1(distanceToTarget) -> horizontalDistance/1  "distanceToTdp"
  LogicController/2(timeHorizontal) -> onTargetTime/1  "timeToHorizontalTDP"
  LogicController/3(timeVertical) -> touchdownTime/1  "timeToVerticalTDP"
  LogicController/6(desiredCourse) -> Scope4/1, Targeting/2(Course2Target)  "courseToTarget"
  Targeting/1(CMD) -> feedback/2(BimCommand), bimCommand/1, Abs/1, Sign/1  "bimCommand"
  Bus Selector/2 -> LogicController/2(currentPoint)  "<ActualPosition>"
  Bus Selector/3 -> LogicController/3(reliefAvailable)  "<ReliefAvailable>"
  Bus Selector/4 -> LogicController/4(reliefc)  "<Relief>"
  Bus Selector/5 -> LogicController/5(reliefOnTDP)  "<ReliefOnTDP>"
  Bus Selector/6 -> LogicController/6(course)  "<Course>"
  Bus Selector1/1 -> feedback/3(TDPoint)  "<TDP>"
  Bus Selector1/2 -> feedback/4(Course)  "<Course>"
  Bus Selector1/3 -> feedback/5(HorizontalSpeed)  "<HorizontalSpeed>"
  feedback/2(BimWasEnabled) -> Bus Creator1/2  "BimWasEnabled"
  feedback/3(BimWasDisabled) -> Bus Creator1/3  "BimWasDisabled"
  Bus Creator1/1 -> Bus Selector2/1, Bus Selector4/1
  Bus Selector2/1 -> LogicController/9(fallingBim)  "<BimWasDisabled>"
  Bus Selector2/2 -> LogicController/10(risingBim)  "<BimWasEnabled>"
  Bus Selector2/3 -> LogicController/11(touchdownPointOffset)  "<TDPofset>"
  Bus Selector3/1 -> Targeting/3(TrackingCourse)  "<Course>"
  feedback/1(PointPopr) -> Bus Creator1/1  "TDPofset"
  Bus Selector/1 -> LogicController/1(touchdownPoint)  "<TDP>"
  BimTimeout/1 -> Data Store Write5/1
  VSpeed/1 -> Data Store Write6/1
  HSpeed/1 -> Data Store Write7/1
  FallingTime/1 -> Data Store Write8/1
  Bus Selector4/1 -> Display/1  "<TDPofset>"
  Bus Creator/1 -> Bus Selector5/1, Bus Selector3/1, Bus Selector1/1, Bus Selector6/1, Bus Selector/1
  Bus Selector5/1 -> Scope/1  "<ReliefAvailable>"
  Bus Selector5/2 -> Scope3/1  "<Relief>"
  Bus Selector5/3 -> Scope5/1  "<ReliefOnTDP>"
  Bus Selector5/4 -> Radians to Degrees/1, Scope6/1  "<Course>"
  Bus Selector5/5 -> Scope7/1  "<HorizontalSpeed>"
  Bus Selector5/6 -> Scope8/1  "<VerticalSpeed>"
  AngleTimeout/1 -> Data Store Write9/1
  Degrees to Radians/1 -> Data Store Write1/1
  LogicController/7(skipOfsetSolution) -> feedback/1(Skip), Scope9/1  "skipOfsetSolution"
  Bus Selector6/1 -> LogicController/7(velocityHorizontal)  "<HorizontalSpeed>"
  Bus Selector6/2 -> LogicController/8(velocityVertical)  "<VerticalSpeed>"
  Sign/1 -> Data Type Conversion/1
  Abs/1 -> Data Type Conversion1/1
  Radians to Degrees/1 -> Scope2/1
  weightCoefficient/1 -> Data Store Write10/1
  Data Type Conversion/1 -> bimSelect/1
  Data Type Conversion1/1 -> bimForce/1
  touchdownPoint/1 -> Demux/1  "TDP"
  Demux/1 -> Bus Creator3/1  "touchdownPoint:latitude"
  Demux/2 -> Bus Creator3/2  "touchdownPoint:longitude"
  Demux/3 -> Bus Creator3/3  "touchdownPoint:atlitude"
  touchdownPointRelief/1 -> Bus Creator3/4  "touchdownPoint:relief"
  radioPoint/1 -> Demux1/1
  radioPointRelief/1 -> Bus Creator4/4  "radioPoint:relief"
  Demux1/3 -> Bus Creator4/3  "radioPoint:altitude"
  Demux1/2 -> Bus Creator4/2  "radioPoint:longitude"
  Demux1/1 -> Bus Creator4/1  "radioPoint:latitude"
  Demux2/3 -> Bus Creator5/3  "currentPoint:altitude"
  currentPoint/1 -> Demux2/1
  currentRelief/1 -> Bus Creator5/4  "currentPoint:relief"
  velocityLatitude/1 -> Bus Creator2/1  "gpsVelocity:latitude"
  velocityLongitude/1 -> Bus Creator2/2  "gpsVelocity:longitude"
  velocityAltitude/1 -> Bus Creator2/3  "gpsVelocity:altitude"
  Bus Creator3/1 -> Bus Creator6/1  "touchdownPoint"
  Bus Creator4/1 -> Bus Creator6/2  "radioPoint"
  Bus Creator5/1 -> Bus Creator6/3  "currentPoint"
  Bus Creator2/1 -> Bus Creator6/4  "gpsVelocity"
  currentReliefAvailable/1 -> Bus Creator6/5  "currentPoint:reliefAvailable"
  trackingCourse/1 -> Bus Creator6/8  "trackingCourse"
  barometricAltitude/1 -> Bus Creator6/6  "barometricAltitude"
  barometricAvailable/1 -> Bus Creator6/7  "barometricAvailable"
  Bus Selector8/1 -> DataAnalyzer/1(ActualPoint)  "<currentPoint>"
  Bus Selector8/2 -> DataAnalyzer/2(ActualCourse)  "<trackingCourse>"
  Bus Creator6/1 -> Bus Creator7/1, Bus Selector12/1, Bus Selector8/1  "input"
  Bus Selector8/3 -> DataAnalyzer/3(Velocity)  "<gpsVelocity>"
  Bus Selector12/1 -> altitudeWeighting/1(gpsPosition)  "<currentPoint>"
  Bus Selector12/2 -> altitudeWeighting/2(barometricAltitude)  "<barometricAltitude>"
  Bus Selector12/3 -> altitudeWeighting/3(barometricAvailable)  "<barometricAvailable>"
  radioUpdateIndex/1 -> Bus Creator6/9  "radioUpdateIndex"
  DataAnalyzer/2(HorizontalVelocity) -> Bus Creator8/1  "velocity:horizontal"
  DataAnalyzer/3(VerticalVelocity) -> Bus Creator8/2  "velocity:vertical"
  Bus Creator8/1 -> Bus Creator7/4  "velocity"
  DataAnalyzer/1(TrackingCourse) -> Bus Creator7/3  "course"
  Demux2/2 -> Bus Creator5/2  "currentPoint:longitude"
  Demux2/1 -> Bus Creator5/1  "currentPoint:latitude"
  altitudeWeighting/1(position) -> Bus Creator7/2
  Bus Creator7/1 -> Bus Creator9/1, Bus Selector7/1  "processData"
  Bus Selector7/1 -> TargetSelector/1(touchdownPoint)  "<touchdownPoint>"
  Bus Selector7/2 -> TargetSelector/2(radioPoint)  "<radioPoint>"
  Bus Selector7/3 -> TargetSelector/3(currentPoint)  "<currentPoint>"
  Bus Selector7/4 -> TargetSelector/4(radioUpdateIndex)  "<radioUpdateIndex>"
  Bus Selector7/5 -> TargetSelector/5(verticalVelocity)  "<velocity:vertical>"
  Bus Selector7/6 -> TargetSelector/6(currentCourse)  "<course>"
  TargetSelector/1(targetPoint) -> Bus Creator9/2
  Bus Creator9/1 -> Bus Selector9/1

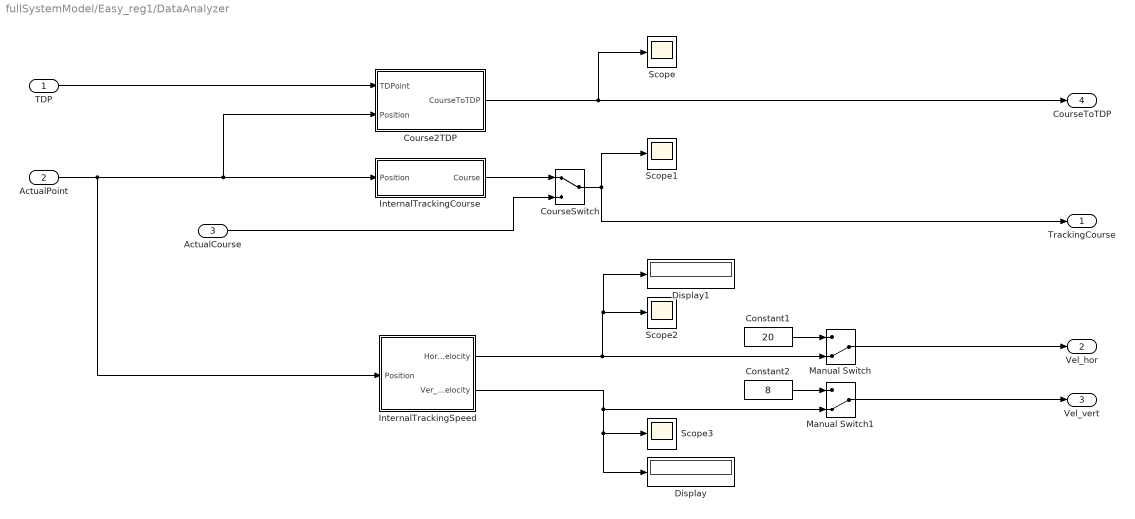
== system fullSystemModel/Easy_reg1/DataAnalyzer ==
  TDP : Inport
  ActualPoint : Inport  Port=2
  ActualCourse : Inport  Port=3
  Constant1 : Constant  Value=20
  Constant2 : Constant  Value=8
  Course2TDP : Subsystem
  CourseSwitch : ManualSwitch
  Display : Display
  Display1 : Display
  InternalTrackingCourse : Subsystem
  InternalTrackingSpeed : Subsystem
  Manual Switch : ManualSwitch  CurrentSetting=0
  Manual Switch1 : ManualSwitch  CurrentSetting=0
  Scope{,1..3} (4 alike) : Scope
  TrackingCourse : Outport
  Vel_hor : Outport  Port=2
  Vel_vert : Outport  Port=3
  CourseToTDP : Outport  Port=4
  wires:
  CourseSwitch/1 -> TrackingCourse/1, Scope1/1
  TDP/1 -> Course2TDP/1(TDPoint)
  InternalTrackingCourse/1(Course) -> CourseSwitch/1
  ActualCourse/1 -> CourseSwitch/2
  ActualPoint/1 -> InternalTrackingSpeed/1(Position), Course2TDP/2(Position), InternalTrackingCourse/1(Position)
  InternalTrackingSpeed/1(Hor_Velocity) -> Manual Switch/2, Display1/1, Scope2/1
  InternalTrackingSpeed/2(Ver_Velocity) -> Manual Switch1/2, Scope3/1, Display/1
  Manual Switch/1 -> Vel_hor/1
  Constant1/1 -> Manual Switch/1
  Manual Switch1/1 -> Vel_vert/1
  Course2TDP/1(CourseToTDP) -> Scope/1, CourseToTDP/1
  Constant2/1 -> Manual Switch1/1

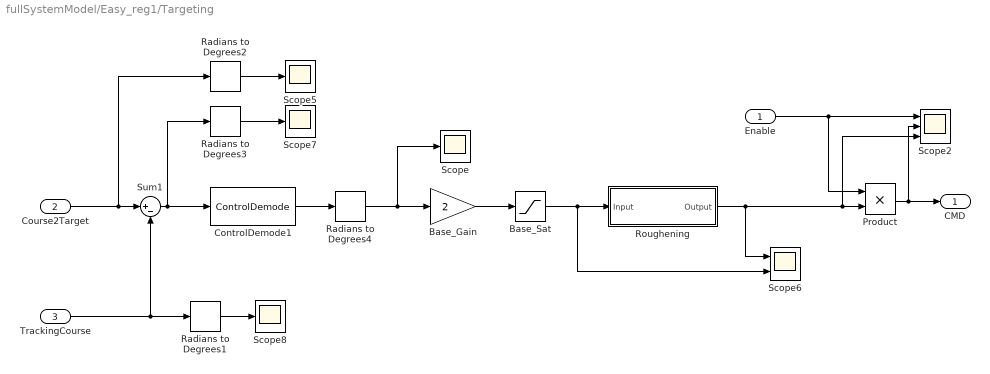
== system fullSystemModel/Easy_reg1/Targeting ==
  Enable : Inport  OutDataTypeStr=uint8  PortDimensions=1
  Course2Target : Inport  Port=2  OutDataTypeStr=double  PortDimensions=1
  TrackingCourse : Inport  Port=3  OutDataTypeStr=double  PortDimensions=1
  Base_Gain : Gain  Gain=2
  Base_Sat : Saturate  UpperLimit=50  LowerLimit=-50
  ControlDemode1 : BupSimulinkLibraries/ControlDemode
  Product : Product
  Radians to Degrees{1..4} (4 alike) : simulink_extras/Transformations/Radians to Degrees
  Roughening : Subsystem
  Scope{,5,7..8} (4 alike) : Scope
  Scope2 : Scope  NumInputPorts=3
  Scope6 : Scope  NumInputPorts=2
  Sum1 : Sum  Inputs=|+-
  CMD : Outport  OutDataTypeStr=double
  wires:
  Course2Target/1 -> Radians to Degrees2/1, Sum1/1
  Radians to Degrees3/1 -> Scope7/1
  Radians to Degrees2/1 -> Scope5/1
  Base_Sat/1 -> Scope6/2, Roughening/1(Input)
  Base_Gain/1 -> Base_Sat/1
  Radians to Degrees4/1 -> Scope/1, Base_Gain/1
  Enable/1 -> Product/1, Scope2/1
  Product/1 -> Scope2/2, CMD/1
  TrackingCourse/1 -> Radians to Degrees1/1, Sum1/2
  Sum1/1 -> ControlDemode1/1, Radians to Degrees3/1
  ControlDemode1/1 -> Radians to Degrees4/1
  Roughening/1(Output) -> Product/2, Scope2/3, Scope6/1
  Radians to Degrees1/1 -> Scope8/1

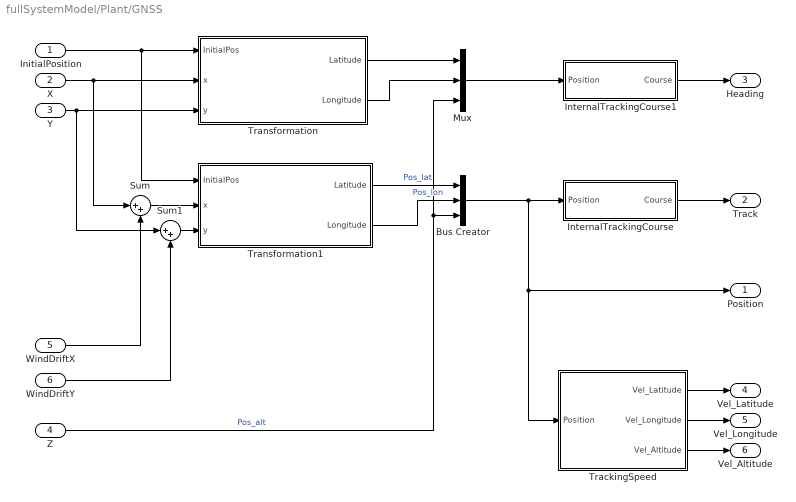
== system fullSystemModel/Plant/GNSS ==
  InitialPosition : Inport
  X : Inport  Port=2
  Y : Inport  Port=3
  Z : Inport  Port=4
  WindDriftX : Inport  Port=5
  WindDriftY : Inport  Port=6
  Bus Creator : BusCreator  Inputs=3
  InternalTrackingCourse : Subsystem
  InternalTrackingCourse1 : Subsystem
  Mux : Mux  Inputs=3
  Sum : Sum  Inputs=|++
  Sum1 : Sum  Inputs=|++
  TrackingSpeed : Subsystem
  Transformation : Subsystem
  Transformation1 : Subsystem
  Position : Outport
  Track : Outport  Port=2
  Heading : Outport  Port=3
  Vel_Latitude : Outport  Port=4
  Vel_Longitude : Outport  Port=5
  Vel_Altitude : Outport  Port=6
  wires:
  InitialPosition/1 -> Transformation1/1(InitialPos), Transformation/1(InitialPos)
  X/1 -> Sum/1, Transformation/2(x)
  Y/1 -> Sum1/1, Transformation/3(y)
  Sum/1 -> Transformation1/2(x)
  Sum1/1 -> Transformation1/3(y)
  WindDriftX/1 -> Sum/2
  WindDriftY/1 -> Sum1/2
  TrackingSpeed/2(Vel_Longitude) -> Vel_Longitude/1
  TrackingSpeed/3(Vel_Altitude) -> Vel_Altitude/1
  TrackingSpeed/1(Vel_Latitude) -> Vel_Latitude/1
  Transformation/1(Latitude) -> Mux/1
  Transformation/2(Longitude) -> Mux/2
  Mux/1 -> InternalTrackingCourse1/1(Position)
  Transformation1/1(Latitude) -> Bus Creator/1  "Pos_lat"
  Bus Creator/1 -> InternalTrackingCourse/1(Position), TrackingSpeed/1(Position), Position/1
  Z/1 -> Mux/3, Bus Creator/3  "Pos_alt"
  InternalTrackingCourse1/1(Course) -> Heading/1
  InternalTrackingCourse/1(Course) -> Track/1
  Transformation1/2(Longitude) -> Bus Creator/2  "Pos_lon"

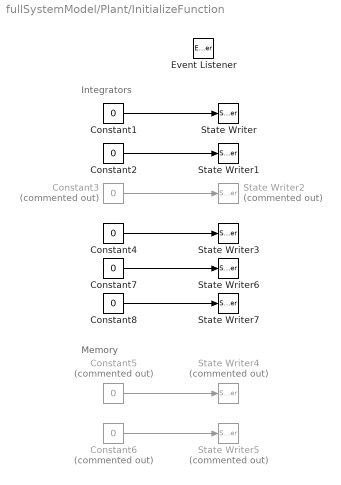
== system fullSystemModel/Plant/InitializeFunction ==
  note: Memory
  note: Integrators
  Constant{1..2,4,7..8} (5 alike) : Constant  Value=0
  Constant3 : Constant  Commented=on  Value=0
  Constant5 : Constant  Commented=on  Value=0
  Constant6 : Constant  Commented=on  Value=0
  Event Listener : EventListener  DisableCoverage=on  EventName=reset
  State Writer : StateWriter  StateOwnerBlock=../../x_integrator
  State Writer1 : StateWriter  StateOwnerBlock=../../y_integrator
  State Writer2 : StateWriter  Commented=on  StateOwnerBlock=../../angle_integrator
  State Writer3 : StateWriter  StateOwnerBlock=../../timer_integrator
  State Writer4 : StateWriter  Commented=on
  State Writer5 : StateWriter  Commented=on
  State Writer6 : StateWriter  StateOwnerBlock=../../WindCreator/WindXintegrator
  State Writer7 : StateWriter  StateOwnerBlock=../../WindCreator/WindYintegrator
  wires:
  Constant1/1 -> State Writer/1
  Constant2/1 -> State Writer1/1
  Constant3/1 -> State Writer2/1
  Constant4/1 -> State Writer3/1
  Constant5/1 -> State Writer4/1
  Constant6/1 -> State Writer5/1
  Constant7/1 -> State Writer6/1
  Constant8/1 -> State Writer7/1

== system fullSystemModel/Plant/ResetFunction ==
  note: Memory
  note: Integrators
  Constant{1..2,4,7..8} (5 alike) : Constant  Value=0
  Constant3 : Constant  Commented=on  Value=0
  Constant5 : Constant  Commented=on  Value=0
  Constant6 : Constant  Commented=on  Value=0
  Event Listener : EventListener  DisableCoverage=on  EventType=Reset  EventName=reset
  State Writer : StateWriter  StateOwnerBlock=../../x_integrator
  State Writer1 : StateWriter  StateOwnerBlock=../../y_integrator
  State Writer2 : StateWriter  Commented=on  StateOwnerBlock=../../angle_integrator
  State Writer3 : StateWriter  StateOwnerBlock=../../timer_integrator
  State Writer4 : StateWriter  Commented=on
  State Writer5 : StateWriter  Commented=on
  State Writer6 : StateWriter  StateOwnerBlock=../../WindCreator/WindXintegrator
  State Writer7 : StateWriter  StateOwnerBlock=../../WindCreator/WindYintegrator
  wires:
  Constant1/1 -> State Writer/1
  Constant2/1 -> State Writer1/1
  Constant3/1 -> State Writer2/1
  Constant4/1 -> State Writer3/1
  Constant5/1 -> State Writer4/1
  Constant6/1 -> State Writer5/1
  Constant7/1 -> State Writer6/1
  Constant8/1 -> State Writer7/1

== system fullSystemModel/Plant/RotateOnNorth ==
  AbsoluteAngle : Inport
  Constant : Constant  Value=90
  Gain : Gain  Gain=-1
  Sum3 : Sum  Inputs=|+-
  OrientedOnNorth : Outport
  wires:
  AbsoluteAngle/1 -> Sum3/1
  Constant/1 -> Sum3/2
  Sum3/1 -> Gain/1
  Gain/1 -> OrientedOnNorth/1

== system fullSystemModel/Plant/SWS ==
  Pos_alt : Inport
  Constant : Constant  Value=20
  Constant1 : Constant  Value=20
  Constant2 : Constant  Value=20
  Sum3 : Sum  Inputs=++|
  Height : Outport
  TrueSpeed : Outport  Port=2
  InstrumentalSpeed : Outport  Port=3
  wires:
  Sum3/1 -> Height/1
  Constant/1 -> Sum3/1
  Pos_alt/1 -> Sum3/2
  Constant1/1 -> TrueSpeed/1
  Constant2/1 -> InstrumentalSpeed/1

== system fullSystemModel/Plant/WindCreator ==
  WindAngle : Inport
  WindSpeed : Inport  Port=2
  Degrees to Radians1 : simulink_extras/Transformations/Degrees to Radians
  Product1 : Product
  Product2 : Product
  RotateOnNorth : Subsystem
  Trigonometric Function2 : Trigonometry  Operator=cos
  Trigonometric Function3 : Trigonometry
  WindXintegrator : DiscreteIntegrator  SampleTime=-1  ICPrevOutput=DiscIntNeverNeededParam  ICPrevScaledInput=DiscIntNeverNeededParam
  WindYintegrator : DiscreteIntegrator  SampleTime=-1  ICPrevOutput=DiscIntNeverNeededParam  ICPrevScaledInput=DiscIntNeverNeededParam
  WindXPos : Outport
  WindYPos : Outport  Port=2
  wires:
  Product1/1 -> WindYintegrator/1
  WindSpeed/1 -> Product1/2, Product2/2
  Trigonometric Function2/1 -> Product2/1
  RotateOnNorth/1(OrientedOnNorth) -> Degrees to Radians1/1
  Trigonometric Function3/1 -> Product1/1
  Degrees to Radians1/1 -> Trigonometric Function3/1, Trigonometric Function2/1
  WindAngle/1 -> RotateOnNorth/1(AbsoluteAngle)
  Product2/1 -> WindXintegrator/1
  WindYintegrator/1 -> WindYPos/1
  WindXintegrator/1 -> WindXPos/1

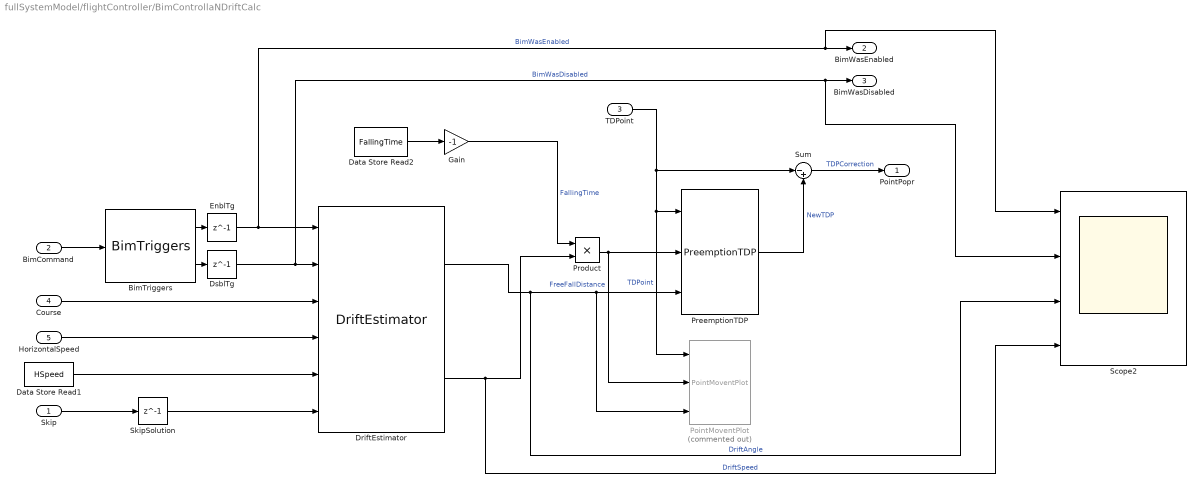
== system fullSystemModel/flightController/BimControllaNDriftCalc ==
  Skip : Inport
  BimCommand : Inport  Port=2
  TDPoint : Inport  Port=3
  Course : Inport  Port=4
  HorizontalSpeed : Inport  Port=5
  BimTriggers : BupSimulinkLibraries/BimTriggers
  Data Store Read1 : DataStoreRead  DataStoreName=HSpeed
  Data Store Read2 : DataStoreRead  DataStoreName=FallingTime
  DriftEstimator : BupSimulinkLibraries/DriftEstimator
  DsblTg : Delay  DelayLength=1  InitialCondition=0
  EnblTg : Delay  DelayLength=1  InitialCondition=0
  Gain : Gain  Gain=-1
  PointMoventPlot : BupSimulinkLibraries/PointMoventPlot  Commented=on
  PreemptionTDP : BupSimulinkLibraries/PreemptionTDP
  Product : Product
  Scope2 : Scope  NumInputPorts=4
  SkipSolution : Delay  DelayLength=1  InitialCondition=0
  Sum : Sum  Inputs=|-+
  PointPopr : Outport
  BimWasEnabled : Outport  Port=2
  BimWasDisabled : Outport  Port=3
  wires:
  PreemptionTDP/1 -> Sum/2  "NewTDP"
  DriftEstimator/2 -> Scope2/4, Product/2  "DriftSpeed"
  BimCommand/1 -> BimTriggers/1
  DriftEstimator/1 -> Scope2/3, PointMoventPlot/3, PreemptionTDP/3  "DriftAngle"
  Data Store Read1/1 -> DriftEstimator/5
  Data Store Read2/1 -> Gain/1
  EnblTg/1 -> Scope2/1, BimWasEnabled/1, DriftEstimator/1  "BimWasEnabled"
  Product/1 -> PointMoventPlot/2, PreemptionTDP/2  "FreeFallDistance"
  TDPoint/1 -> Sum/1, PointMoventPlot/1, PreemptionTDP/1  "TDPoint"
  BimTriggers/2 -> DsblTg/1
  BimTriggers/1 -> EnblTg/1
  HorizontalSpeed/1 -> DriftEstimator/4
  Course/1 -> DriftEstimator/3
  DsblTg/1 -> Scope2/2, BimWasDisabled/1, DriftEstimator/2  "BimWasDisabled"
  Sum/1 -> PointPopr/1  "TDPCorrection"
  Gain/1 -> Product/1  "FallingTime"
  Skip/1 -> SkipSolution/1
  SkipSolution/1 -> DriftEstimator/6

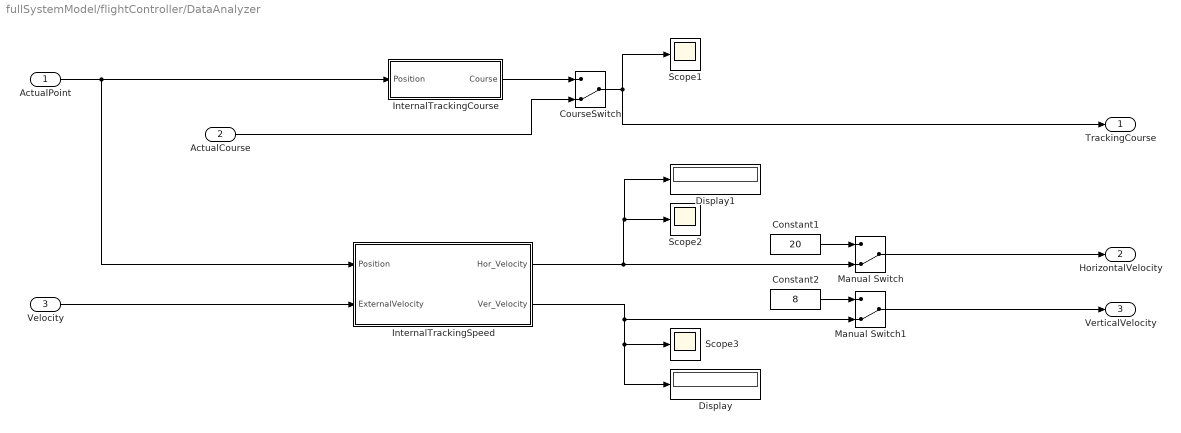
== system fullSystemModel/flightController/DataAnalyzer ==
  ActualPoint : Inport
  ActualCourse : Inport  Port=2
  Velocity : Inport  Port=3
  Constant1 : Constant  Value=20
  Constant2 : Constant  Value=8
  CourseSwitch : ManualSwitch  CurrentSetting=0
  Display : Display
  Display1 : Display
  InternalTrackingCourse : Subsystem
  InternalTrackingSpeed : Subsystem
  Manual Switch : ManualSwitch  CurrentSetting=0
  Manual Switch1 : ManualSwitch  CurrentSetting=0
  Scope1 : Scope
  Scope2 : Scope
  Scope3 : Scope
  TrackingCourse : Outport
  HorizontalVelocity : Outport  Port=2
  VerticalVelocity : Outport  Port=3
  wires:
  CourseSwitch/1 -> TrackingCourse/1, Scope1/1
  InternalTrackingCourse/1(Course) -> CourseSwitch/1
  ActualCourse/1 -> CourseSwitch/2
  ActualPoint/1 -> InternalTrackingSpeed/1(Position), InternalTrackingCourse/1(Position)
  InternalTrackingSpeed/1(Hor_Velocity) -> Manual Switch/2, Display1/1, Scope2/1
  InternalTrackingSpeed/2(Ver_Velocity) -> Manual Switch1/2, Scope3/1, Display/1
  Manual Switch/1 -> HorizontalVelocity/1
  Constant1/1 -> Manual Switch/1
  Manual Switch1/1 -> VerticalVelocity/1
  Constant2/1 -> Manual Switch1/1
  Velocity/1 -> InternalTrackingSpeed/2(ExternalVelocity)

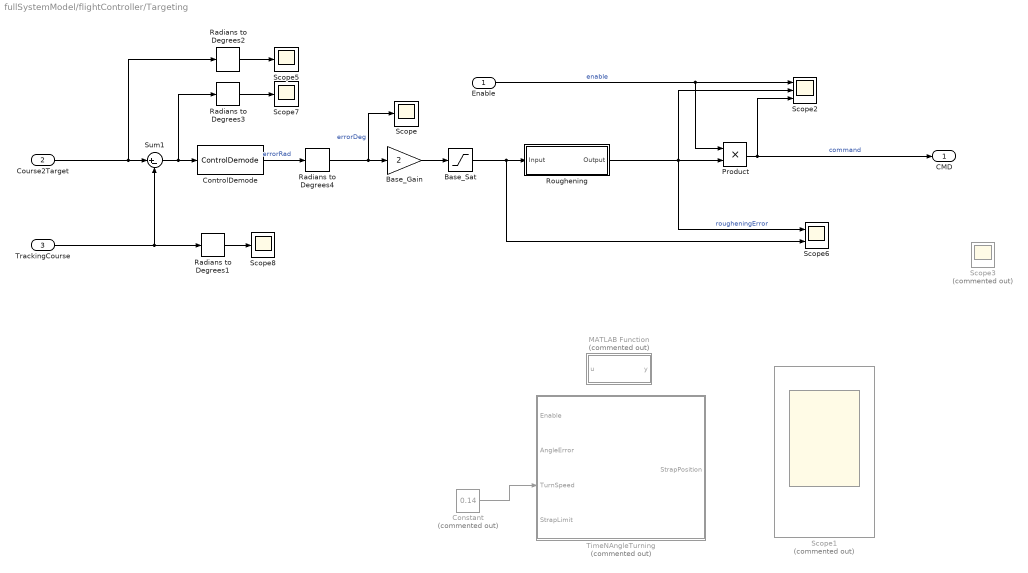
== system fullSystemModel/flightController/Targeting ==
  Enable : Inport  OutDataTypeStr=uint8  PortDimensions=1
  Course2Target : Inport  Port=2  OutDataTypeStr=double  PortDimensions=1
  TrackingCourse : Inport  Port=3  OutDataTypeStr=double  PortDimensions=1
  Base_Gain : Gain  Gain=2
  Base_Sat : Saturate  UpperLimit=50  LowerLimit=-50
  Constant : Constant  Commented=on  Value=0.14
  ControlDemode : BupSimulinkLibraries/ControlDemode
  MATLAB Function : MATLAB Function  Commented=on  TreatAsAtomicUnit=on
  Product : Product
  Radians to Degrees{1..4} (4 alike) : simulink_extras/Transformations/Radians to Degrees
  Roughening : Subsystem
  Scope{,5,7..8} (4 alike) : Scope
  Scope1 : Scope  Commented=on  NumInputPorts=4
  Scope2 : Scope  NumInputPorts=3
  Scope3 : Scope  Commented=on  NumInputPorts=2
  Scope6 : Scope  NumInputPorts=2
  Sum1 : Sum  Inputs=|+-
  TimeNAngleTurning : Stateflow chart  Commented=on  TreatAsAtomicUnit=on  SystemSampleTime=1
  CMD : Outport  OutDataTypeStr=double
  wires:
  Course2Target/1 -> Sum1/1, Radians to Degrees2/1
  Radians to Degrees3/1 -> Scope7/1
  Radians to Degrees2/1 -> Scope5/1
  Base_Gain/1 -> Base_Sat/1
  Radians to Degrees4/1 -> Scope/1, Base_Gain/1  "errorDeg"
  Enable/1 -> Product/1, Scope2/1  "enable"
  Product/1 -> Scope2/3, CMD/1  "command"
  TrackingCourse/1 -> Radians to Degrees1/1, Sum1/2
  Sum1/1 -> ControlDemode/1, Radians to Degrees3/1
  ControlDemode/1 -> Radians to Degrees4/1  "errorRad"
  Roughening/1(Output) -> Scope2/2, Product/2, Scope6/1  "rougheningError"
  Radians to Degrees1/1 -> Scope8/1
  Base_Sat/1 -> Scope6/2, Roughening/1(Input)
  Constant/1 -> TimeNAngleTurning/3(TurnSpeed)

== system fullSystemModel/flightController/altitudeWeighting ==
  gpsPosition : Inport
  barometricAltitude : Inport  Port=2
  barometricAvailable : Inport  Port=3  OutMin=[0]  OutMax=[1]  OutDataTypeStr=uint8  PortDimensions=1
  Add : Sum
  Bus Creator3 : BusCreator  Inputs=4
  Bus Selector1 : BusSelector  OutputSignals=currentPoint:latitude,currentPoint:longitude,currentPoint:relief
  Bus Selector7 : BusSelector  OutputSignals=currentPoint:altitude
  Data Store Read2 : DataStoreRead  DataStoreName=AltitudeWeight
  Product : Product
  Product1 : Product
  Scope : Scope
  Sum : Sum  Inputs=|-+
  Switch : Switch  Criteria=u2 > Threshold
  constant : Constant
  position : Outport
  wires:
  Product/1 -> Add/2
  Add/1 -> Bus Creator3/3, Scope/1  "currentPoint:altitude"
  Product1/1 -> Add/1
  Sum/1 -> Product/1
  Data Store Read2/1 -> Product1/2, Sum/1
  Bus Selector7/1 -> Product1/1  "<currentPoint:altitude>"
  gpsPosition/1 -> Bus Selector1/1, Bus Selector7/1, Switch/3
  constant/1 -> Sum/2
  barometricAvailable/1 -> Switch/2
  Bus Creator3/1 -> Switch/1
  barometricAltitude/1 -> Product/2
  Switch/1 -> position/1  "currentPoint"
  Bus Selector1/1 -> Bus Creator3/1  "<currentPoint:latitude>"
  Bus Selector1/2 -> Bus Creator3/2  "<currentPoint:longitude>"
  Bus Selector1/3 -> Bus Creator3/4  "<currentPoint:relief>"

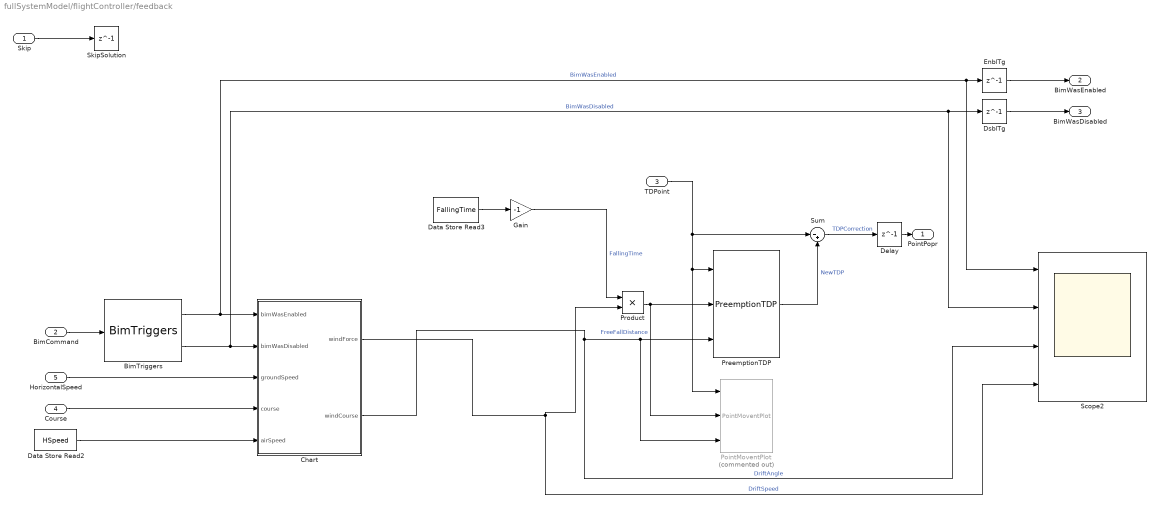
== system fullSystemModel/flightController/feedback ==
  Skip : Inport
  BimCommand : Inport  Port=2
  TDPoint : Inport  Port=3
  Course : Inport  Port=4
  HorizontalSpeed : Inport  Port=5
  BimTriggers : BupSimulinkLibraries/BimTriggers
  Chart : Stateflow chart  TreatAsAtomicUnit=on
  Data Store Read2 : DataStoreRead  DataStoreName=HSpeed
  Data Store Read3 : DataStoreRead  DataStoreName=FallingTime
  Delay : Delay  DelayLength=1  InitialCondition=0
  DsblTg : Delay  DelayLength=1  InitialCondition=0
  EnblTg : Delay  DelayLength=1  InitialCondition=0
  Gain : Gain  Gain=-1
  PointMoventPlot : BupSimulinkLibraries/PointMoventPlot  Commented=on
  PreemptionTDP : BupSimulinkLibraries/PreemptionTDP
  Product : Product
  Scope2 : Scope  NumInputPorts=4
  SkipSolution : Delay  DelayLength=1  InitialCondition=0
  Sum : Sum  Inputs=|-+
  PointPopr : Outport
  BimWasEnabled : Outport  Port=2
  BimWasDisabled : Outport  Port=3
  wires:
  Gain/1 -> Product/1  "FallingTime"
  TDPoint/1 -> Sum/1, PointMoventPlot/1, PreemptionTDP/1
  Chart/2(windCourse) -> Scope2/3, PointMoventPlot/3, PreemptionTDP/3  "DriftAngle"
  Skip/1 -> SkipSolution/1
  Product/1 -> PointMoventPlot/2, PreemptionTDP/2  "FreeFallDistance"
  Sum/1 -> Delay/1  "TDPCorrection"
  PreemptionTDP/1 -> Sum/2  "NewTDP"
  Data Store Read3/1 -> Gain/1
  BimCommand/1 -> BimTriggers/1
  Chart/1(windForce) -> Product/2, Scope2/4  "DriftSpeed"
  BimTriggers/1 -> Chart/1(bimWasEnabled), Scope2/1, EnblTg/1  "BimWasEnabled"
  BimTriggers/2 -> Scope2/2, DsblTg/1, Chart/2(bimWasDisabled)  "BimWasDisabled"
  EnblTg/1 -> BimWasEnabled/1
  DsblTg/1 -> BimWasDisabled/1
  Course/1 -> Chart/4(course)
  HorizontalSpeed/1 -> Chart/3(groundSpeed)
  Data Store Read2/1 -> Chart/5(airSpeed)
  Delay/1 -> PointPopr/1

== system fullSystemModel/Easy_reg1/DataAnalyzer/Course2TDP ==
  TDPoint : Inport
  Position : Inport  Port=2
  Bearing : BupSimulinkLibraries/Bearing
  CourseToTDP : Outport
  wires:
  Position/1 -> Bearing/2
  TDPoint/1 -> Bearing/1
  Bearing/1 -> CourseToTDP/1
